simulink model "rameno_2D"  (R2023a)
settings: Solver=VariableStepAuto  StartTime=0.0  StopTime=2.4  MaxStep=0.001  RelTol=1e-3  AbsTol=1e-3  EnableMultiTasking=on
InitFcn:
  | data;
values from neighbouring files (symbols this model uses):
  akt = [0,1,0,0,0,0,0,0]    [data.m]    (also in optim_control_nlmpc.m = u'; reaction_angle.m = u)
  coords = [params.GHsx params.GHsy params.GHhx params. GHhy]    [data.m]    (also in optim_control_nlmpc.m; optim_control_optimtraj.m)
  koef = [params.ms params.mh params.Is params.Ih params.g params.c]    [data.m]    (also in optim_control_nlmpc.m; optim_control_optimtraj.m)
  x0 = [-0.03904,0.1411925,0,0]    [data.m]
undefined symbols (not defined in the file or in its folder): muscles, params, X, Y, Z
libraries: sm_lib x54, nesl_utility x23
(part 2 of 2)

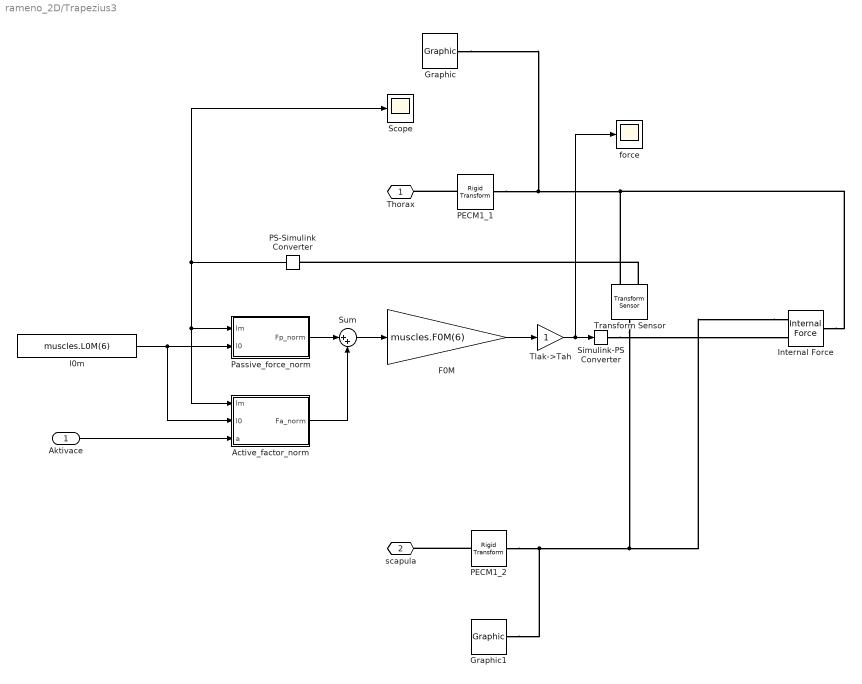
== system rameno_2D/Trapezius3 ==
  Aktivace : Inport
  Active_factor_norm : MATLAB Function  TreatAsAtomicUnit=on
  F0M : Gain  Gain=muscles.F0M(6)
  Graphic : sm_lib/Body Elements/Graphic  GraphicType=Marker  MarkerShape=Sphere  MarkerSize=10  GraphicVisPropType=SimpleVisualProperties  GraphicDiffuseColor=[0 1 1]  GraphicSpecularColor=[0.5 0.5 0.5 1.0]  GraphicAmbientColor=[0.15 0.15 0.15 1.0]  GraphicEmissiveColor=[0.0 0.0 0.0 1.0]  GraphicShininess=75  GraphicOpacity=1.0
  Graphic1 : sm_lib/Body Elements/Graphic  GraphicType=Marker  MarkerShape=Sphere  MarkerSize=10  GraphicVisPropType=SimpleVisualProperties  GraphicDiffuseColor=[0.05882 1 1]  GraphicSpecularColor=[0.5 0.5 0.5 1.0]  GraphicAmbientColor=[0.15 0.15 0.15 1.0]  GraphicEmissiveColor=[0.0 0.0 0.0 1.0]  GraphicShininess=75  GraphicOpacity=1.0
  Internal Force : sm_lib/Forces and Torques/Internal Force
  PECM1_1 : sm_lib/Frames and Transforms/Rigid Transform  TranslationMethod=Cartesian  TranslationStandardOffset=0  TranslationStandardOffsetUnits=m  TranslationStandardAxis=+Z  TranslationCartesianOffset=[muscles.origin(6,:),0]  TranslationCartesianOffsetUnits=m  TranslationROffset=0  TranslationROffsetUnits=m  TranslationZOffset=0  TranslationZOffsetUnits=m  TranslationThetaOffset=0  TranslationThetaOffsetUnits=deg  RotationMethod=None  RotationAngleUnits=deg  RotationStandardAxis=+Z  RotationAngle=0.0  RotationArbitraryAxis=[0 0 1]  FollAlignAxisA=+X  BaseAlignAxisA=+Y  FollAlignAxisB=+Y  BaseAlignAxisB=+Z  RotationSequenceAxes=FollowerAxes  RotationSequence=XYX  RotationSequenceAngles=[0 0 0]  RotationSequenceAnglesUnits=deg  RotationMatrix=[1 0 0; 0 1 0; 0 0 1]  Quaternion=[1 0 0 0]
  PECM1_2 : sm_lib/Frames and Transforms/Rigid Transform  TranslationMethod=Cartesian  TranslationStandardOffset=0  TranslationStandardOffsetUnits=m  TranslationStandardAxis=+Z  TranslationCartesianOffset=[muscles.insertion(6,:),0]  TranslationCartesianOffsetUnits=m  TranslationROffset=0  TranslationROffsetUnits=m  TranslationZOffset=0  TranslationZOffsetUnits=m  TranslationThetaOffset=0  TranslationThetaOffsetUnits=deg  RotationMethod=None  RotationAngleUnits=deg  RotationStandardAxis=+Y  RotationAngle=90  RotationArbitraryAxis=[0 0 1]  FollAlignAxisA=+X  BaseAlignAxisA=+Y  FollAlignAxisB=+Y  BaseAlignAxisB=+Z  RotationSequenceAxes=FollowerAxes  RotationSequence=XYX  RotationSequenceAngles=[0 0 0]  RotationSequenceAnglesUnits=deg  RotationMatrix=[1 0 0; 0 1 0; 0 0 1]  Quaternion=[1 0 0 0]
  PS-Simulink Converter : nesl_utility/PS-Simulink Converter  PhysicalDomain=network_engine_domain  SubClassName=ps_output  LeftPortType=input  RightPortType=output  PseudoPeriodic=off  Frequencies=[]  VectorFormat=inherit  Unit=inherit  AffineConversion=off
  Passive_force_norm : MATLAB Function  TreatAsAtomicUnit=on
  Scope : Scope
  Simulink-PS Converter : nesl_utility/Simulink-PS Converter  PhysicalDomain=network_engine_domain  SubClassName=ps_input  LeftPortType=input  RightPortType=output  PseudoPeriodic=off  Frequencies=[]  NoiseDistribution=none  NoiseParameters=[]  Unit=1  AffineConversion=off  FilteringAndDerivatives=provide  SimscapeFilterOrder=1  InputFilterTimeConstant=0.001  UdotUserProvided=0
  Sum : Sum  Inputs=|++
  Tlak->Tah : Gain
  Transform Sensor : sm_lib/Frames and Transforms/Transform Sensor  MeasurementFrame=World  RotationSequence=XYX  SenseAngle=off  SenseAxis=off  SenseQ=off  SenseR=off  SenseRotationSequence=off  SenseOmegaX=off  SenseOmegaY=off  SenseOmegaZ=off  SenseQDot=off  SenseRDot=off  SenseRotationSequenceDot=off  SenseAlphaX=off  SenseAlphaY=off  SenseAlphaZ=off  SenseQDDot=off  SenseRDDot=off  SenseX=off  SenseY=off  SenseZ=off  SenseRad=off  SenseAzim=off  SenseDist=on  SenseInc=off  SenseXDot=off  SenseYDot=off  SenseZDot=off  SenseRadDot=off  SenseAzimDot=off  SenseDistDot=off  SenseIncDot=off  SenseXDDot=off  SenseYDDot=off  SenseZDDot=off  SenseRadDDot=off  SenseAzimDDot=off  SenseDistDDot=off  SenseIncDDot=off
  force : Scope
  l0m : Constant  Value=muscles.L0M(6)
  Thorax : PMIOPort  Side=Left
  scapula : PMIOPort  Port=2  Side=Left
  wires:
  Sum/1 -> F0M/1
  F0M/1 -> Tlak->Tah/1
  Passive_force_norm/1(Fp_norm) -> Sum/1
  Active_factor_norm/1(Fa_norm) -> Sum/2
  Tlak->Tah/1 -> Simulink-PS Converter/1, force/1
  PS-Simulink Converter/1 -> Scope/1, Active_factor_norm/1(lm), Passive_force_norm/1(lm)
  l0m/1 -> Active_factor_norm/2(l0), Passive_force_norm/2(l0)
  Aktivace/1 -> Active_factor_norm/3(a)
  connections:
  Internal Force/LConn1 -- Transform Sensor/LConn1 -- Graphic1/RConn1 -- PECM1_2/RConn1
  Internal Force/RConn1 -- PECM1_1/RConn1 -- Graphic/RConn1 -- Transform Sensor/RConn1
  Simulink-PS Converter/RConn1 -- Internal Force/LConn2
  Transform Sensor/RConn2 -- PS-Simulink Converter/LConn1
  PECM1_1/LConn1 -- Thorax/RConn1
  PECM1_2/LConn1 -- scapula/RConn1

== matlab function rameno_2D/Trapezius2/Active_factor_norm ==
  data: Fa_norm output; lm input; l0 input; a input
function Fa_norm = fcn(lm,l0,a)
f_gauss = 0.25;
Fa_norm = (exp(-(lm/l0-1)^2/f_gauss))*a;

== matlab function rameno_2D/Trapezius2/Passive_force_norm ==
  data: lm input; Fp_norm output; l0 input
function Fp_norm = fcn(lm,l0)
Fp_norm = ((lm/l0)^3)*exp(8*lm/l0-12.9);

== matlab function rameno_2D/MATLAB Function1 ==
  data: u input; y output
function y = fcn(u)
y = zeros(3,1);
y = [30;atan(u(2)/u(1))*180/pi;-30];

== matlab function rameno_2D/DELT/Active_factor_norm ==
  data: Fa_norm output; lm input; l0 input; a input
function Fa_norm = fcn(lm,l0,a)
f_gauss = 0.25;
Fa_norm = (exp(-(lm/l0-1)^2/f_gauss))*a;

== matlab function rameno_2D/DELT/Passive_force_norm ==
  data: lm input; Fp_norm output; l0 input
function Fp_norm = fcn(lm,l0)
Fp_norm = ((lm/l0)^3)*exp(8*lm/l0-12.9);

== matlab function rameno_2D/DELT/MATLAB Function ==
  data: u input; length output
function length = muscle_length(u)
O_posit = [0.05, 0.035];
I_posit = [0.01,0.05];
GHsx = 0.075;
GHsy = 0.0028;
GHhx = 0;
GHhy = 0.1;
O = position(O_posit(1),O_posit(2));
I = T_x(GHsx)*T_y(GHsy)*R_z(u)*T_x(-GHhx)*T_y(-GHhy)*position(I_posit(1),I_posit(2));
centre = [GHsx,GHsy,1];
radius = 0.02;
length = muscle_length_wrap(O',I',centre,radius);

function trans_x = T_x(x)
    trans_x = [1,0,x;
               0,1,0;
               0,0,1];
end

function trans_y = T_y(y)
    trans_y = [1,0,0;
               0,1,y;
               0,0,1];
end


function rot_phiz = R_z(phiz)
    rot_phiz = [cos(phiz),-sin(phiz),0;
                sin(phiz), cos(phiz),0;
                0           ,0      ,1];
end

function r = position(x,y)
    r = [x;y;1];
end

function len = muscle_length_wrap(origin,insertion,centre,radius)
    wrap_len = wrap_angle(origin,insertion,centre,radius)*radius;
    I_pos = wrap_point(insertion,centre,radius,1);
    O_pos = wrap_point(origin,centre,radius,-1);
    O_len = vec_dist(O_pos,origin);
    I_len = vec_dist(I_pos,insertion);
    len = wrap_len+O_len+I_len;
end

function len = vec_dist(O,I)
    len = sqrt((O(1) - I(1))^2 + (O(2) - I(2))^2);
end

function angle = wrap_angle(origin,insertion,centre,radius)
    O_pos = wrap_point(origin,centre,radius,-1);
    I_pos = wrap_point(insertion,centre,radius,1);
    angle =  atan2(O_pos(2)-centre(2),O_pos(1)-centre(1))-atan2(I_pos(2)-centre(2),I_pos(1)-centre(1));
end

function pos = wrap_point(attach,centre,radius,direction)
    side = [0,0,1]+centre;
    attach_f = att_frame(attach, centre, side);
    base = norm(attach-centre);
    x = radius^2/base;
    y = direction*sqrt(radius^2-x^2);
    % angle = vecangle360(x_cyl,attach_f,side);
    angle = atan2(attach_f(2),attach_f(1));
    pos = T_x(centre(1))*T_y(centre(2))*R_z(angle)*[x;y;1];
end

function x_ax = att_frame(attach, centre, side)
    z_ax = (side-centre)/norm(side-centre);
    y_ax = cross(z_ax,attach-centre)/norm(cross(z_ax,attach-centre));
    x_ax = cross(y_ax,z_ax);
end
end

== matlab function rameno_2D/Supraspinatus/Active_factor_norm ==
  data: Fa_norm output; lm input; l0 input; a input
function Fa_norm = fcn(lm,l0,a)
f_gauss = 0.25;
Fa_norm = (exp(-(lm/l0-1)^2/f_gauss))*a;

== matlab function rameno_2D/Supraspinatus/Passive_force_norm ==
  data: lm input; Fp_norm output; l0 input
function Fp_norm = fcn(lm,l0)
Fp_norm = ((lm/l0)^3)*exp(8*lm/l0-12.9);

== matlab function rameno_2D/Trapezius3/Active_factor_norm ==
  data: Fa_norm output; lm input; l0 input; a input
function Fa_norm = fcn(lm,l0,a)
f_gauss = 0.25;
Fa_norm = (exp(-(lm/l0-1)^2/f_gauss))*a;

== matlab function rameno_2D/Trapezius3/Passive_force_norm ==
  data: lm input; Fp_norm output; l0 input
function Fp_norm = fcn(lm,l0)
Fp_norm = ((lm/l0)^3)*exp(8*lm/l0-12.9);

== matlab function rameno_2D/Rhomboideus/Active_factor_norm ==
  data: Fa_norm output; lm input; l0 input; a input
function Fa_norm = fcn(lm,l0,a)
f_gauss = 0.25;
Fa_norm = (exp(-(lm/l0-1)^2/f_gauss))*a;

== matlab function rameno_2D/Rhomboideus/Passive_force_norm ==
  data: lm input; Fp_norm output; l0 input
function Fp_norm = fcn(lm,l0)
Fp_norm = ((lm/l0)^3)*exp(8*lm/l0-12.9);

== matlab function rameno_2D/reakce ==
  data: x1 input size=1; dx1 input size=1; ddx1 input; R output; x2 input size=1; dx2 input size=1; ddx2 input; acc output; akt input; angle output
function [R,acc,angle] = fcn(x1,dx1,ddx1,x2,dx2,ddx2,akt)
x = zeros(1,4);
R = 0;
acc = 0;
% zrychleni jako kdyby bylo vynasobeno rotacni matici inverzni, 
x = [x1,x2,dx1,dx2];
% R = reactions(x1,dx1,ddx1,x2,dx2,ddx2,GHsx,GHsy,GHhx,GHhy,g,mh,origin,insertion, O_pos, I_pos,l0m,force,akt);
% angle = reaction_angle(x',akt);
angle = phi_react(x,akt');
% acc = [GHhx.*(ddx1.*sin(x1 + x2) + ddx2.*sin(x1 + x2) + dx1.^2.*cos(x1 + x2) + 2*dx1.*dx2.*cos(x1 + x2) + dx2.^2.*cos(x1 + x2)) - GHhy.*(-ddx1.*cos(x1 + x2) - ddx2.*cos(x1 + x2) + dx1.^2.*sin(x1 + x2) + 2*dx1.*dx2.*sin(x1 + x2) + dx2.^2.*sin(x1 + x2)) - GHsx.*ddx1.*sin(x1) - GHsx.*dx1.^2.*cos(x1) - GHsy.*ddx1.*cos(x1) + GHsy.*dx1.^2.*sin(x1); GHhx.*(-ddx1.*cos(x1 + x2) - ddx2.*cos(x1 + x2) + dx1.^2.*sin(x1 + x2) + 2*dx1.*dx2.*sin(x1 + x2) + dx2.^2.*sin(x1 + x2)) + GHhy.*(ddx1.*sin(x1 + x2) + ddx2.*sin(x1 + x2) + dx1.^2.*cos(x1 + x2) + 2*dx1.*dx2.*cos(x1 + x2) + dx2.^2.*cos(x1 + x2)) + GHsx.*ddx1.*cos(x1) - GHsx.*dx1.^2.*sin(x1) - GHsy.*ddx1.*sin(x1) - GHsy.*dx1.^2.*cos(x1); 0];

== matlab function rameno_2D/MATLAB Function ==
  data: t input; dy output; y input; koef parameter; coords parameter; akt input
function dy = fcn(t,y,koef, coords,akt)
dy = zeros(4,1);
% dy = ODE_sim(t,y,koef,coords,force,l0m,akt);
force = [450.0;700.0;400.0;700.0;600.0;800.0;300.0;600.1]'*(-1);
l0m = [0.11;0.11;0.08;0.165;0.14;0.14;0.13;0.12]';
mm = MM(t,y,koef,coords,force,l0m,akt');
fo = FO(t,y,koef,coords,force,l0m,akt');
fe = FE(t,y,koef,coords,force,l0m,akt');
dy = real(mm\(fo+fe));

== matlab function rameno_2D/Levator/Active_factor_norm ==
  data: Fa_norm output; lm input; l0 input; a input
function Fa_norm = fcn(lm,l0,a)
f_gauss = 0.25;
Fa_norm = (exp(-(lm/l0-1)^2/f_gauss))*a;

== matlab function rameno_2D/Levator/Passive_force_norm ==
  data: lm input; Fp_norm output; l0 input
function Fp_norm = fcn(lm,l0)
Fp_norm = ((lm/l0)^3)*exp(8*lm/l0-12.9);

== matlab function rameno_2D/TerMin/Active_factor_norm ==
  data: Fa_norm output; lm input; l0 input; a input
function Fa_norm = fcn(lm,l0,a)
f_gauss = 0.25;
Fa_norm = (exp(-(lm/l0-1)^2/f_gauss))*a;

== matlab function rameno_2D/TerMin/Passive_force_norm ==
  data: lm input; Fp_norm output; l0 input
function Fp_norm = fcn(lm,l0)
Fp_norm = ((lm/l0)^3)*exp(8*lm/l0-12.9);

== matlab function rameno_2D/Trapezius1/Active_factor_norm ==
  data: Fa_norm output; lm input; l0 input; a input
function Fa_norm = fcn(lm,l0,a)
f_gauss = 0.25;
Fa_norm = (exp(-(lm/l0-1)^2/f_gauss))*a;

== matlab function rameno_2D/Trapezius1/Passive_force_norm ==
  data: lm input; Fp_norm output; l0 input
function Fp_norm = fcn(lm,l0)
Fp_norm = ((lm/l0)^3)*exp(8*lm/l0-12.9);
